simulink library "tqr"  (R2021b)
settings: Solver=VariableStepAuto  StartTime=0.0  StopTime=10.0  RelTol=1e-3
undefined symbols (not defined in the file or in its folder): ATQR_AltRDCActiveFEDUInc_X_pct, ATQR_AltRDCActiveFEDUInc_Y_enum, ATQR_AltRDCActiveFEDUTs_X_pct, ATQR_AltRDCActiveFEDUTs_Y_enum, ATQR_AltRDCActiveREDUInc_X_pct, ATQR_AltRDCActiveREDUInc_Y_enum, ATQR_AltRDCActiveREDUTs_X_pct, ATQR_AltRDCActiveREDUTs_Y_enum, ATQR_CreepFEDUTqIncSR_X_rpm, ATQR_CreepFEDUTqIncSR_Y_Nm, ATQR_CreepFEDUTs_X_rpm, ATQR_CreepFEDUTs_Y_Nm, ATQR_EcoTqFrIncGain_X_Nm, ATQR_EcoTqFrIncGain_Y_pct, ATQR_EcoTqRrIncGain_X_Nm, ATQR_EcoTqRrIncGain_Y_pct, ATQR_EL1FEDUTqDecSR_Y_Nm, ATQR_EL1FEDUTqIncSR_X_rpm, ATQR_EL1FEDUTqIncSR_Y_pct, ATQR_EL1FEDUTs_X_rpm, ATQR_EL1FEDUTs_Y_Nm, ATQR_EL1REDUTqDecSR_Y_Nm, ATQR_EL1REDUTs_Y_Nm, ATQR_FEDUEL1RegenTs_X_rpm, ATQR_FEDUTIPOutTs_X_rpm, ATQR_FrNegRateLimitIncN_X_rpm, ATQR_FrNegRateLimitIncN_Y_Nm, ATQR_FrPosRateLimitIncN_X_rpm, ATQR_FrPosRateLimitIncN_Y_Nm, ATQR_FShaftSpdTqLimCoe_X_rpm, ATQR_FTimerTqLimCoe_X_s, ATQR_FTqZeroTransUpBoundN_X_rpm, ATQR_NL1FEDUTqDecSR_Y_Nm, ATQR_NL1FEDUTqIncSR_X_rpm, ATQR_NL1FEDUTqIncSR_Y_pct, ATQR_NL1FEDUTs_X_rpm, ATQR_NL1FEDUTs_Y_Nm, ATQR_NL1REDUTqDecSR_Y_Nm, ATQR_NL1REDUTs_Y_Nm, ATQR_NormalTqFrIncGain_X_Nm, ATQR_NormalTqFrIncGain_Y_pct, ATQR_NormalTqRrIncGain_X_Nm, ATQR_NormalTqRrIncGain_Y_pct, ATQR_RrNegRateLimitIncN_X_rpm, ATQR_RrNegRateLimitIncN_Y_Nm, ATQR_RrPosRateLimitIncN_X_rpm, ATQR_RrPosRateLimitIncN_Y_Nm, ATQR_RShaftSpdTqLimCoe_X_rpm, ATQR_RTimerTqLimCoe_X_s, ATQR_SL1FEDUTqDecSR_Y_Nm, ATQR_SL1FEDUTqIncSR_X_rpm, ATQR_SL1FEDUTqIncSR_Y_pct, ATQR_SL1FEDUTs_X_rpm, ATQR_SL1FEDUTs_Y_Nm, ATQR_SL1REDUTqDecSR_Y_Nm, ATQR_SL1REDUTs_Y_Nm, ATQR_SportTqFrIncGain_X_Nm, ATQR_SportTqFrIncGain_Y_pct, ATQR_SportTqRrIncGain_X_Nm, ATQR_SportTqRrIncGain_Y_pct ... (+269)
libraries: hcu_lib x15, simulink x13, $bdroot x3
(part 3 of 9)

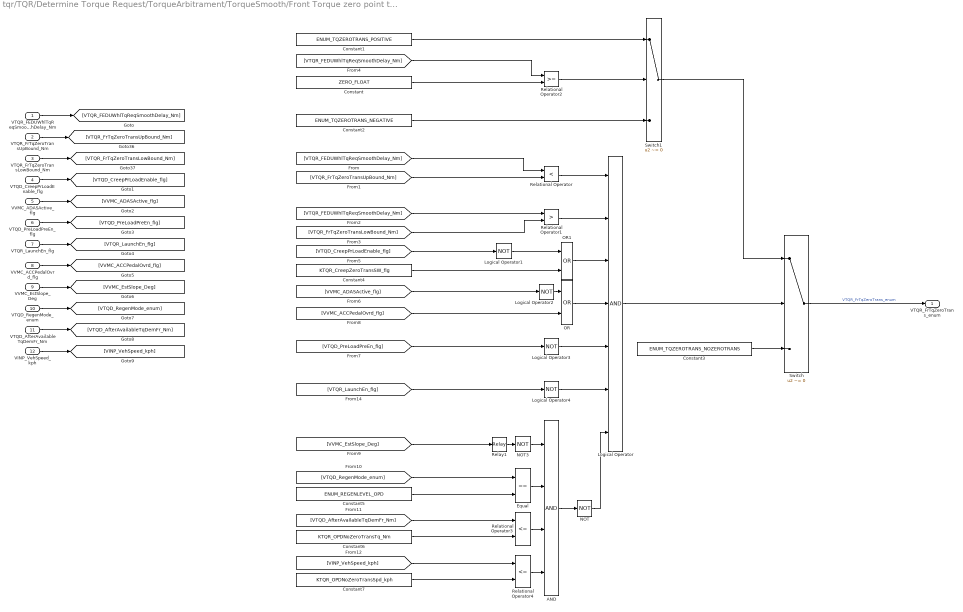
== system tqr/TQR/Determine Torque Request/TorqueArbitrament/TorqueSmooth/Front Torque zero point transfer status determination  ==
  VTQR_FEDUWhlTqReqSmoothDelay_Nm : Inport
  VTQR_FrTqZeroTransUpBound_Nm : Inport  Port=2
  VTQR_FrTqZeroTransLowBound_Nm : Inport  Port=3
  VTQD_CreepPrLoadEnable_flg : Inport  Port=4
  VVMC_ADASActive_flg : Inport  Port=5
  VTQD_PreLoadPreEn_flg : Inport  Port=6
  VTQR_LaunchEn_flg : Inport  Port=7
  VVMC_ACCPedalOvrd_flg : Inport  Port=8
  VVMC_EstSlope_Deg : Inport  Port=9
  VTQD_RegenMode_enum : Inport  Port=10
  VTQD_AfterAvailableTqDemFr_Nm : Inport  Port=11
  VINP_VehSpeed_kph : Inport  Port=12
  AND : Logic  Inputs=4  AllPortsSameDT=off  OutDataTypeStr=boolean
  Constant : Constant  Value=ZERO_FLOAT
  Constant1 : Constant  Value=ENUM_TQZEROTRANS_POSITIVE
  Constant2 : Constant  Value=ENUM_TQZEROTRANS_NEGATIVE
  Constant3 : Constant  Value=ENUM_TQZEROTRANS_NOZEROTRANS
  Constant4 : Constant  Value=KTQR_CreepZeroTransSW_flg
  Constant5 : Constant  Value=ENUM_REGENLEVEL_OPD
  Constant6 : Constant  Value=KTQR_OPDNoZeroTransTq_Nm
  Constant7 : Constant  Value=KTQR_OPDNoZeroTransSpd_kph
  Equal : RelationalOperator  Operator===  OutDataTypeStr=boolean  RndMeth=Simplest
  Logical Operator : Logic  Inputs=7  AllPortsSameDT=off  OutDataTypeStr=boolean
  Logical Operator{1..4} (4 alike) : Logic  Operator=NOT  AllPortsSameDT=off  OutDataTypeStr=boolean
  NOT : Logic  Operator=NOT  AllPortsSameDT=off  OutDataTypeStr=boolean
  NOT3 : Logic  Operator=NOT  AllPortsSameDT=off  OutDataTypeStr=boolean
  OR : Logic  Operator=OR  AllPortsSameDT=off  OutDataTypeStr=boolean
  OR1 : Logic  Operator=OR  AllPortsSameDT=off  OutDataTypeStr=boolean
  Relational Operator : RelationalOperator  Operator=<  OutDataTypeStr=boolean  RndMeth=Simplest
  Relational Operator1 : RelationalOperator  Operator=>  OutDataTypeStr=boolean  RndMeth=Simplest
  Relational Operator2 : RelationalOperator  OutDataTypeStr=boolean  RndMeth=Simplest
  Relational Operator3 : RelationalOperator  Operator=<=  OutDataTypeStr=boolean  RndMeth=Simplest
  Relational Operator4 : RelationalOperator  Operator=<=  OutDataTypeStr=boolean  RndMeth=Simplest
  Relay1 : Relay  OnSwitchValue=KTQD_OPDHoldGradeUp_Deg  OffSwitchValue=KTQD_OPDHoldGradeDown_Deg  OutDataTypeStr=boolean
  Switch : Switch  Criteria=u2 ~= 0
  Switch1 : Switch  Criteria=u2 ~= 0
  VTQR_FrTqZeroTrans_enum : Outport
  wires:
  VTQR_FEDUWhlTqReqSmoothDelay_Nm/1 -> [VTQR_FEDUWhlTqReqSmoothDelay_Nm]
  VTQR_FrTqZeroTransUpBound_Nm/1 -> [VTQR_FrTqZeroTransUpBound_Nm]
  VTQR_FrTqZeroTransLowBound_Nm/1 -> [VTQR_FrTqZeroTransLowBound_Nm]
  VTQD_CreepPrLoadEnable_flg/1 -> [VTQD_CreepPrLoadEnable_flg]
  VVMC_ADASActive_flg/1 -> [VVMC_ADASActive_flg]
  VTQD_PreLoadPreEn_flg/1 -> [VTQD_PreLoadPreEn_flg]
  VTQR_LaunchEn_flg/1 -> [VTQR_LaunchEn_flg]
  VVMC_ACCPedalOvrd_flg/1 -> [VVMC_ACCPedalOvrd_flg]
  Logical Operator2/1 -> OR/1
  [VTQR_LaunchEn_flg] -> Logical Operator4/1
  Relational Operator1/1 -> Logical Operator/2
  Relational Operator2/1 -> Switch1/2
  [VTQR_FrTqZeroTransLowBound_Nm] -> Relational Operator1/2
  OR/1 -> Logical Operator/4
  [VVMC_ACCPedalOvrd_flg] -> OR/2
  Logical Operator/1 -> Switch/2
  Logical Operator4/1 -> Logical Operator/6
  [VTQR_FEDUWhlTqReqSmoothDelay_Nm] -> Relational Operator2/1
  [VVMC_ADASActive_flg] -> Logical Operator2/1
  Switch1/1 -> Switch/1
  Logical Operator3/1 -> Logical Operator/5
  [VTQR_FEDUWhlTqReqSmoothDelay_Nm] -> Relational Operator/1
  Constant3/1 -> Switch/3
  [VTQD_PreLoadPreEn_flg] -> Logical Operator3/1
  [VTQD_CreepPrLoadEnable_flg] -> Logical Operator1/1
  Constant2/1 -> Switch1/3
  Constant1/1 -> Switch1/1
  Relational Operator/1 -> Logical Operator/1
  [VTQR_FrTqZeroTransUpBound_Nm] -> Relational Operator/2
  [VTQR_FEDUWhlTqReqSmoothDelay_Nm] -> Relational Operator1/1
  Constant/1 -> Relational Operator2/2
  Switch/1 -> VTQR_FrTqZeroTrans_enum/1  "VTQR_FrTqZeroTrans_enum"
  OR1/1 -> Logical Operator/3
  Logical Operator1/1 -> OR1/1
  Constant4/1 -> OR1/2
  Constant6/1 -> Relational Operator3/2
  NOT3/1 -> AND/1
  Constant7/1 -> Relational Operator4/2
  NOT/1 -> Logical Operator/7
  Relay1/1 -> NOT3/1
  Relational Operator3/1 -> AND/3
  Relational Operator4/1 -> AND/4
  Equal/1 -> AND/2
  Constant5/1 -> Equal/2
  AND/1 -> NOT/1
  [VVMC_EstSlope_Deg] -> Relay1/1
  [VTQD_RegenMode_enum] -> Equal/1
  [VTQD_AfterAvailableTqDemFr_Nm] -> Relational Operator3/1
  [VINP_VehSpeed_kph] -> Relational Operator4/1
  VINP_VehSpeed_kph/1 -> [VINP_VehSpeed_kph]
  VTQD_AfterAvailableTqDemFr_Nm/1 -> [VTQD_AfterAvailableTqDemFr_Nm]
  VTQD_RegenMode_enum/1 -> [VTQD_RegenMode_enum]
  VVMC_EstSlope_Deg/1 -> [VVMC_EstSlope_Deg]

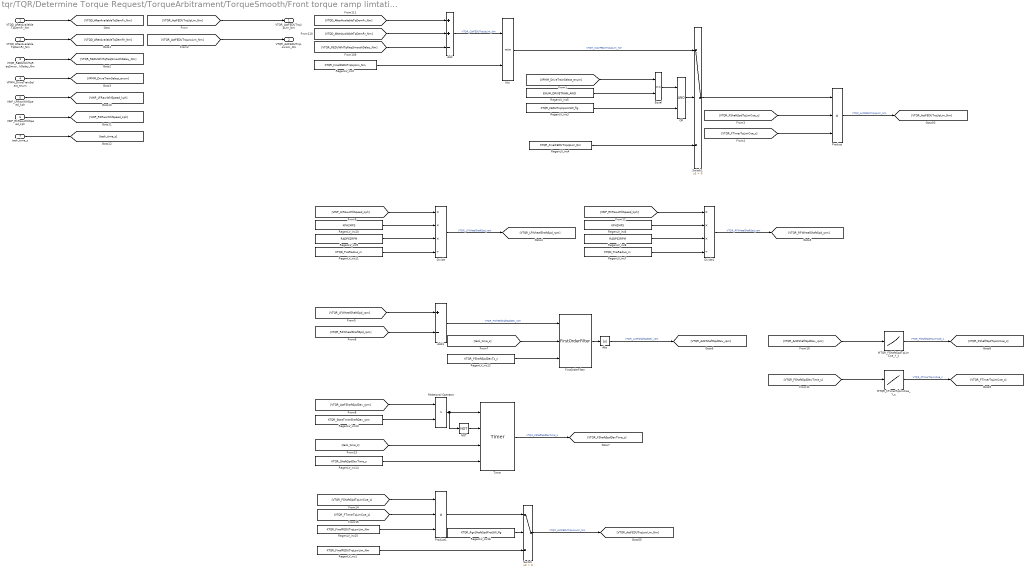
== system tqr/TQR/Determine Torque Request/TorqueArbitrament/TorqueSmooth/Front torque ramp limtation and determination ==
  VTQD_AfterAvailableTqDemFr_Nm : Inport
  VTQD_AfterAvailableTqDemRr_Nm : Inport  Port=2
  VTQR_REDUWhlTqReqSmoothDelay_Nm : Inport  Port=3
  VPMM_DriveTrainSelect_enum : Inport  Port=4
  VINP_LFRawWhlSpeed_kph : Inport  Port=5
  VINP_RFRawWhlSpeed_kph : Inport  Port=6
  task_time_s : Inport  Port=7
  Abs : Abs
  Add : Sum  Inputs=++-
  Add1 : Sum  Inputs=+-
  Divide : Product  Inputs=***/
  Divide1 : Product  Inputs=***/
  Equal : RelationalOperator  Operator===  OutDataTypeStr=boolean  RndMeth=Simplest
  FirstOrderFilter : hcu_lib/Basic_Blocks/FirstOrderFilter
  MTQR_FShaftSpdTqLimCoe_Y_c : Lookup_n-D  NumberOfTableDimensions=1  BreakpointsForDimension1=ATQR_FShaftSpdTqLimCoe_X_rpm  Table=MTQR_FShaftSpdTqLimCoe_Y_c  InternalRulePriority=Speed  RndMeth=Simplest  InputSameDT=on
  MTQR_FTimerTqLimCoe_Y_c : Lookup_n-D  NumberOfTableDimensions=1  BreakpointsForDimension1=ATQR_FTimerTqLimCoe_X_s  Table=MTQR_FTimerTqLimCoe_Y_c  InternalRulePriority=Speed  RndMeth=Simplest  InputSameDT=on
  Min : MinMax  Inputs=2
  NOT : Logic  Operator=NOT  AllPortsSameDT=off  OutDataTypeStr=boolean
  OR : Logic  AllPortsSameDT=off  OutDataTypeStr=boolean
  Product : Product  Inputs=3
  Product1 : Product  Inputs=3
  RegenLV_inc1 : Constant  Value=KTQR_FinalFEDUTrqLowLim_Nm  OutDataTypeStr=single
  RegenLV_inc10 : Constant  Value=KPH2MPS  OutDataTypeStr=single
  RegenLV_inc11 : Constant  Value=KTQD_TireRadius_m  OutDataTypeStr=single
  RegenLV_inc12 : Constant  Value=KTQR_FShaftSpdDevTs_c  OutDataTypeStr=single
  RegenLV_inc13 : Constant  Value=KTQR_StartTimerShaftDev_rpm  OutDataTypeStr=single
  RegenLV_inc14 : Constant  Value=KTQR_ShaftSpdDevTime_s  OutDataTypeStr=single
  RegenLV_inc15 : Constant  Value=KTQR_FinalFEDUTrqLowLim_Nm  OutDataTypeStr=single
  RegenLV_inc16 : Constant  Value=KTQR_RgnShaftSpdProtSW_flg  OutDataTypeStr=single
  RegenLV_inc2 : Constant  Value=KTQR_FinalFEDUTrqUpLim_Nm  OutDataTypeStr=single
  RegenLV_inc3 : Constant  Value=KTQR_FEDUTrqUpLimSW_flg  OutDataTypeStr=single
  RegenLV_inc4 : Constant  Value=KTQR_FinalFEDUTrqUpLim_Nm  OutDataTypeStr=single
  RegenLV_inc5 : Constant  Value=ENUM_DRIVETRAIN_AWD  OutDataTypeStr=single
  RegenLV_inc6 : Constant  Value=KPH2MPS  OutDataTypeStr=single
  RegenLV_inc7 : Constant  Value=KTQD_TireRadius_m  OutDataTypeStr=single
  RegenLV_inc8 : Constant  Value=RADPS2RPM  OutDataTypeStr=single
  RegenLV_inc9 : Constant  Value=RADPS2RPM  OutDataTypeStr=single
  Relational Operator : RelationalOperator  Operator=>  OutDataTypeStr=boolean  RndMeth=Simplest
  Switch : Switch  Criteria=u2 > Threshold
  Switch1 : Switch  Criteria=u2 > Threshold
  Timer : hcu_lib/Basic_Blocks/Timer
  VTQR_ActFEDUTrqUpLim_Nm : Outport
  VTQR_ActFEDUTrqLowLim_Nm : Outport  Port=2
  wires:
  Add/1 -> Min/1  "VTQR_CalFEDUTrqUpLim_Nm"
  RegenLV_inc2/1 -> Min/2
  Min/1 -> Switch1/1  "VTQR_CoorFEDUTrqUpLim_Nm"
  [VTQD_AfterAvailableTqDemFr_Nm] -> Add/1
  [VTQD_AfterAvailableTqDemRr_Nm] -> Add/2
  RegenLV_inc4/1 -> Switch1/3
  VTQD_AfterAvailableTqDemFr_Nm/1 -> [VTQD_AfterAvailableTqDemFr_Nm]
  VTQD_AfterAvailableTqDemRr_Nm/1 -> [VTQD_AfterAvailableTqDemRr_Nm]
  VTQR_REDUWhlTqReqSmoothDelay_Nm/1 -> [VTQR_REDUWhlTqReqSmoothDelay_Nm]
  VPMM_DriveTrainSelect_enum/1 -> [VPMM_DriveTrainSelect_enum]
  [VTQR_REDUWhlTqReqSmoothDelay_Nm] -> Add/3
  [VTQR_ActFEDUTrqLowLim_Nm] -> VTQR_ActFEDUTrqLowLim_Nm/1
  [VTQR_ActFEDUTrqUpLim_Nm] -> VTQR_ActFEDUTrqUpLim_Nm/1
  [VPMM_DriveTrainSelect_enum] -> Equal/1
  RegenLV_inc5/1 -> Equal/2
  RegenLV_inc3/1 -> OR/2
  OR/1 -> Switch1/2
  Equal/1 -> OR/1
  [VTQR_FShaftSpdDevTime_s] -> MTQR_FTimerTqLimCoe_Y_c/1
  MTQR_FTimerTqLimCoe_Y_c/1 -> [VTQR_FTimerTqLimCoe_c]  "VTQR_FTimerTqLimCoe_c"
  Timer/1 -> [VTQR_FShaftSpdDevTime_s]  "VTQR_FShaftSpdDevTime_s"
  [VTQR_RFWheelShaftSpd_rpm] -> Add1/2
  [VTQR_ActFShaftSpdDev_rpm] -> Relational Operator/1
  Relational Operator/1 -> Timer/1, NOT/1
  MTQR_FShaftSpdTqLimCoe_Y_c/1 -> [VTQR_FShaftSpdTqLimCoe_c]  "VTQR_FShaftSpdTqLimCoe_c"
  RegenLV_inc12/1 -> FirstOrderFilter/3
  RegenLV_inc14/1 -> Timer/4
  [task_time_s] -> Timer/3
  RegenLV_inc9/1 -> Divide/3
  RegenLV_inc6/1 -> Divide1/2
  RegenLV_inc10/1 -> Divide/2
  RegenLV_inc13/1 -> Relational Operator/2
  RegenLV_inc8/1 -> Divide1/3
  [VTQR_ActFShaftSpdDev_rpm] -> MTQR_FShaftSpdTqLimCoe_Y_c/1
  Divide/1 -> [VTQR_LFWheelShaftSpd_rpm]  "VTQR_LFWheelShaftSpd_rpm"
  RegenLV_inc7/1 -> Divide1/4
  Divide1/1 -> [VTQR_RFWheelShaftSpd_rpm]  "VTQR_RFWheelShaftSpd_rpm"
  RegenLV_inc11/1 -> Divide/4
  Add1/1 -> FirstOrderFilter/1  "VTQR_FWheelShaftSpdDev_rpm"
  NOT/1 -> Timer/2
  [VTQR_LFWheelShaftSpd_rpm] -> Add1/1
  [task_time_s] -> FirstOrderFilter/2
  Abs/1 -> [VTQR_ActFShaftSpdDev_rpm]  "VTQR_ActFShaftSpdDev_rpm"
  FirstOrderFilter/1 -> Abs/1
  [VINP_LFRawWhlSpeed_kph] -> Divide/1
  [VINP_RFRawWhlSpeed_kph] -> Divide1/1
  VINP_RFRawWhlSpeed_kph/1 -> [VINP_RFRawWhlSpeed_kph]
  task_time_s/1 -> [task_time_s]
  VINP_LFRawWhlSpeed_kph/1 -> [VINP_LFRawWhlSpeed_kph]
  Switch1/1 -> Product/1
  [VTQR_FTimerTqLimCoe_c] -> Product/3
  [VTQR_FShaftSpdTqLimCoe_c] -> Product/2
  Product/1 -> [VTQR_ActFEDUTrqUpLim_Nm]  "VTQR_ActFEDUTrqUpLim_Nm"
  Product1/1 -> Switch/1
  RegenLV_inc16/1 -> Switch/2
  RegenLV_inc1/1 -> Switch/3
  Switch/1 -> [VTQR_ActFEDUTrqLowLim_Nm]  "VTQR_ActFEDUTrqLowLim_Nm"
  RegenLV_inc15/1 -> Product1/3
  [VTQR_FShaftSpdTqLimCoe_c] -> Product1/1
  [VTQR_FTimerTqLimCoe_c] -> Product1/2

== system tqr/TQR/Determine Torque Request/TorqueArbitrament/TorqueSmooth/Front wheel first order filter input torque command determination ==
  VTQR_FrTqZeroTrans_enum : Inport
  VTQR_FrTqZeroTransUpBound_Nm : Inport  Port=2
  VTQR_FrTqZeroTransLowBound_Nm : Inport  Port=3
  VTQD_AfterAvailableTqDemFr_Nm : Inport  Port=4
  VTQR_FrFirstOrderOutTqDelay_Nm : Inport  Port=5
  VTQR_FrGearChange_flg : Inport  Port=6
  VTQR_RampTqCMDGain_c : Inport  Port=7
  AND : Logic  AllPortsSameDT=off  OutDataTypeStr=boolean
  Constant1 : Constant  Value=ZERO_FLOAT
  Constant2 : Constant  Value=KTQR_GearChangeTqSW_flg
  Constant3 : Constant  Value=ENUM_TQZEROTRANS_NOZEROTRANS
  Constant4 : Constant  Value=KTQR_NewRampArchSW_flg
  Constant5 : Constant  Value=ONE_FLOAT
  Product : Product
  Relational Operator : RelationalOperator  Operator===  OutDataTypeStr=boolean  RndMeth=Simplest
  Relational Operator1 : RelationalOperator  OutDataTypeStr=boolean  RndMeth=Simplest
  Relational Operator2 : RelationalOperator  Operator=<=  OutDataTypeStr=boolean  RndMeth=Simplest
  Switch : Switch  Criteria=u2 ~= 0
  Switch1 : Switch  Criteria=u2 ~= 0
  Switch2 : Switch  Criteria=u2 ~= 0
  Switch3 : Switch  Criteria=u2 > Threshold
  Switch4 : Switch  Criteria=u2 > Threshold
  VTQR_FrFirstOrderInpTq_Nm : Outport
  wires:
  [VTQR_FrTqZeroTrans_enum] -> Relational Operator/1
  Constant3/1 -> Relational Operator/2
  Relational Operator/1 -> Switch/2
  Switch1/1 -> Switch/3
  Relational Operator1/1 -> Switch1/2
  [VTQR_FrFirstOrderOutTqDelay_Nm] -> Relational Operator1/1
  [VTQR_FrTqZeroTransUpBound_Nm] -> Relational Operator1/2
  [VTQR_FrTqZeroTransUpBound_Nm] -> Switch1/1
  Switch3/1 -> VTQR_FrFirstOrderInpTq_Nm/1  "VTQR_FrFirstOrderInpTq_Nm"
  [VTQR_FrTqZeroTransLowBound_Nm] -> Switch2/1
  Switch2/1 -> Switch1/3
  [VTQR_FrFirstOrderOutTqDelay_Nm] -> Relational Operator2/1
  [VTQR_FrTqZeroTransLowBound_Nm] -> Relational Operator2/2
  Relational Operator2/1 -> Switch2/2
  [VTQR_FrActRampTqDem_Nm] -> Switch2/3
  VTQR_FrTqZeroTransLowBound_Nm/1 -> [VTQR_FrTqZeroTransLowBound_Nm]
  VTQR_FrTqZeroTrans_enum/1 -> [VTQR_FrTqZeroTrans_enum]
  VTQR_FrFirstOrderOutTqDelay_Nm/1 -> [VTQR_FrFirstOrderOutTqDelay_Nm]
  VTQD_AfterAvailableTqDemFr_Nm/1 -> [VTQD_AfterAvailableTqDemFr_Nm]
  VTQR_FrTqZeroTransUpBound_Nm/1 -> [VTQR_FrTqZeroTransUpBound_Nm]
  VTQR_FrGearChange_flg/1 -> [VTQR_FrGearChange_flg]
  Constant1/1 -> Switch3/1
  Constant2/1 -> AND/2
  [VTQR_FrGearChange_flg] -> AND/1
  AND/1 -> Switch3/2
  Switch/1 -> Switch3/3
  VTQR_RampTqCMDGain_c/1 -> [VTQR_RampTqCMDGain_c]
  Switch4/1 -> Product/2
  [VTQR_RampTqCMDGain_c] -> Switch4/1
  Constant4/1 -> Switch4/2
  Constant5/1 -> Switch4/3
  Product/1 -> [VTQR_FrActRampTqDem_Nm]  "VTQR_FrActRampTqDem_Nm"
  [VTQR_FrActRampTqDem_Nm] -> Switch/1
  [VTQD_AfterAvailableTqDemFr_Nm] -> Product/1

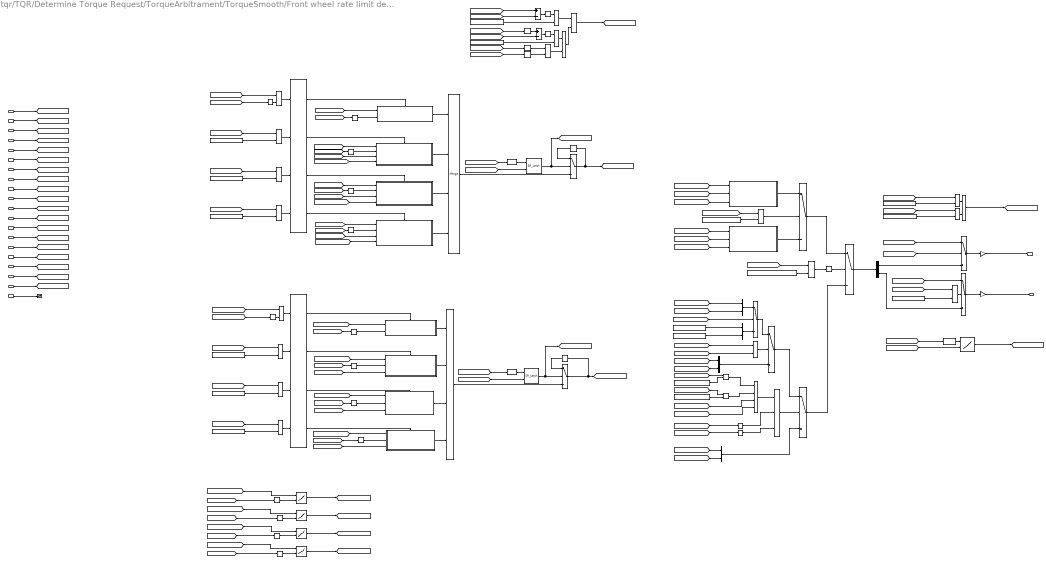
== system tqr/TQR/Determine Torque Request/TorqueArbitrament/TorqueSmooth/Front wheel rate limit determination ==
  VTQR_FrTqZeroTrans_enum : Inport
  VTQD_TqSourceFr_enum : Inport  Port=2
  VTQD_TqTargetShaftSpd_rpm : Inport  Port=3
  VTQD_LimpHomeAct_flg : Inport  Port=4
  VTQR_EVDriveMode_enum : Inport  Port=5
  VDHP_ActAPSPosn_pct : Inport  Port=6
  VTQR_FEDUWhlTqReqSmoothDelay_Nm : Inport  Port=7
  VTQD_EVDriveModeValid_flg : Inport  Port=8
  VTQD_RegenMode_enum : Inport  Port=9
  VVMC_ACCPedalOvrd_flg : Inport  Port=10
  VVMC_CCPedalOvrd_flg : Inport  Port=11
  VTQD_CreepPrLoadEnable_flg : Inport  Port=12
  VTQD_RegenTqLimitEn_flg : Inport  Port=13
  VTQD_RDCActive_enum : Inport  Port=14
  VTQD_PreLoadPreEn_flg : Inport  Port=15
  VTQR_NoABSFEDUWhlTqReq_Nm : Inport  Port=16
  VTQR_RampFEDUWhlTqReq_Nm : Inport  Port=17
  VTQR_FrFirstOrderInpTq_Nm : Inport  Port=18
  VVMC_ActMaxSlideRate_pct : Inport  Port=19
  VTQD_PedAccTqEn_flg : Inport  Port=20
  AND : Logic  AllPortsSameDT=off  OutDataTypeStr=boolean
  AND1 : Logic  Inputs=3  AllPortsSameDT=off  OutDataTypeStr=boolean
  AND2 : Logic  AllPortsSameDT=off  OutDataTypeStr=boolean
  AND4 : Logic  AllPortsSameDT=off  OutDataTypeStr=boolean
  Abs{,1..4,10..13,15..17,43,47} (14 alike) : Abs
  Add : Sum  Inputs=+-
  Add1 : Sum  Inputs=+-
  Constant1 : Constant  Value=ENUM_TQZEROTRANS_NOZEROTRANS
  Constant10 : Constant  Value=KTQR_PreLoadTqIncSR_Nm
  Constant11 : Constant  Value=KTQR_DriveModeCMDTqDev_Nm
  Constant12 : Constant  Value=KTQR_ARegenLatchEnTq_Nm
  Constant13 : Constant  Value=KTQR_PreLoadTqDecSR_Nm
  Constant14 : Constant  Value=ENUM_DRIVEMODE_ECO
  Constant15 : Constant  Value=ENUM_DRIVEMODE_NRM
  Constant17 : Constant  Value=ENUM_DRIVEMODE_SPORT
  Constant2 : Constant  Value=ENUM_RDCACTSTA_NOREQUEST
  Constant3 : Constant  Value=ENUM_TQSOURCE_CC
  Constant34 : Constant  Value=ENUM_TQSOURCE_ADAS
  Constant4 : Constant  Value=ENUM_TQZEROTRANS_POSITIVE
  Constant5 : Constant  Value=KTQR_DriveModeChangeTq_Nm
  Constant6 : Constant  Value=KTQR_RegenTqLimitDecSW_flg
  Constant7 : Constant  Value=ENUM_DRIVEMODE_ECO
  Constant8 : Constant  Value=ENUM_DRIVEMODE_NRM
  Constant9 : Constant  Value=ENUM_DRIVEMODE_SPORT
  Data Type Conversion : DataTypeConversion  OutDataTypeStr=single
  Delay{,1..4} (5 alike) : Delay  DelayLength=1
  Demux : Demux  Outputs=2
  Detect Change : simulink/Logic and Bit Operations/Detect Change  vinit=0  OutDataTypeStr=boolean
  Detect Change1 : simulink/Logic and Bit Operations/Detect Change  vinit=0  OutDataTypeStr=boolean
  Equal{5..6,8,12..13,15} (6 alike) : RelationalOperator  Operator===  OutDataTypeStr=boolean  RndMeth=Simplest
  Equal2 : RelationalOperator  Operator=~=  OutDataTypeStr=boolean  RndMeth=Simplest
  Gain : Gain
  Gain1 : Gain
  If1 : If  NumInputs=4  IfExpression=u1~= 0  ElseIfExpressions=u2 ~= 0, u3 ~= 0,u4 ~= 0  ShowElse=off
  If2 : If  NumInputs=4  IfExpression=u1~= 0  ElseIfExpressions=u2 ~= 0, u3 ~= 0,u4 ~= 0  ShowElse=off
  Logical Operator1 : Logic  Operator=NOT  AllPortsSameDT=off  OutDataTypeStr=boolean
  Logical Operator14 : Logic  Operator=OR  Inputs=4  AllPortsSameDT=off  OutDataTypeStr=boolean
  Logical Operator4 : Logic  Operator=OR  AllPortsSameDT=off  OutDataTypeStr=boolean
  Logical Operator5 : Logic  Operator=NOT  AllPortsSameDT=off  OutDataTypeStr=boolean
  Logical Operator6 : Logic  Operator=OR  AllPortsSameDT=off  OutDataTypeStr=boolean
  Logical Operator7 : Logic  Operator=NOT  AllPortsSameDT=off  OutDataTypeStr=boolean
  MTQR_AltRDCActiveFEDUInc_Z_Nm : Lookup_n-D  BreakpointsForDimension1=ATQR_AltRDCActiveFEDUInc_Y_enum  BreakpointsForDimension2=ATQR_AltRDCActiveFEDUInc_X_pct  Table=MTQR_AltRDCActiveFEDUInc_Z_Nm  TableDataTypeStr=Inherit: Inherit from 'Table data'  ExtrapMethod=Clip  InternalRulePriority=Speed  RndMeth=Simplest  InputSameDT=on
      settings: InputPortMap=u0,u1
  MTQR_CreepFEDUTqDecSR_Z_Nm : Lookup_n-D  BreakpointsForDimension1=ATQR_CreepFEDUTqIncSR_Y_Nm  BreakpointsForDimension2=ATQR_CreepFEDUTqIncSR_X_rpm  Table=MTQR_CreepFEDUTqDecSR_Z_Nm  ExtrapMethod=Clip  InternalRulePriority=Speed  RndMeth=Simplest  InputSameDT=on
      settings: InputPortMap=u0,u1
  MTQR_CreepFEDUTqIncSR_Z_Nm : Lookup_n-D  BreakpointsForDimension1=ATQR_CreepFEDUTqIncSR_Y_Nm  BreakpointsForDimension2=ATQR_CreepFEDUTqIncSR_X_rpm  Table=MTQR_CreepFEDUTqIncSR_Z_Nm  ExtrapMethod=Clip  InternalRulePriority=Speed  RndMeth=Simplest  InputSameDT=on
      settings: InputPortMap=u0,u1
  MTQR_VMCFEDUTqDecSR_Z_Nm : Lookup_n-D  BreakpointsForDimension1=ATQR_VMCFEDUTqIncSR_Y_Nm  BreakpointsForDimension2=ATQR_VMCFEDUTqIncSR_X_rpm  Table=MTQR_VMCFEDUTqDecSR_Z_Nm  ExtrapMethod=Clip  InternalRulePriority=Speed  RndMeth=Simplest  InputSameDT=on
      settings: InputPortMap=u0,u1
  MTQR_VMCFEDUTqIncSR_Z_Nm : Lookup_n-D  BreakpointsForDimension1=ATQR_VMCFEDUTqIncSR_Y_Nm  BreakpointsForDimension2=ATQR_VMCFEDUTqIncSR_X_rpm  Table=MTQR_VMCFEDUTqIncSR_Z_Nm  ExtrapMethod=Clip  InternalRulePriority=Speed  RndMeth=Simplest  InputSameDT=on
      settings: InputPortMap=u0,u1
  Merge1 : Merge  Inputs=4
  Merge2 : Merge  Inputs=4
  Mux{1..4} (4 alike) : Mux  Inputs=2
  NOT : Logic  Operator=NOT  AllPortsSameDT=off  OutDataTypeStr=boolean
  NOT1 : Logic  Operator=NOT  AllPortsSameDT=off  OutDataTypeStr=boolean
  Negative Rate limit Determination : Subsystem  TreatAsAtomicUnit=on
  OR : Logic  Operator=OR  AllPortsSameDT=off  OutDataTypeStr=boolean
  OR2 : Logic  Operator=OR  AllPortsSameDT=off  OutDataTypeStr=boolean
  OR3 : Logic  Operator=OR  AllPortsSameDT=off  OutDataTypeStr=boolean
  Positive Rate limit Determination : Subsystem  TreatAsAtomicUnit=on
  Relational Operator{,1,3..4} (4 alike) : RelationalOperator  Operator===  OutDataTypeStr=boolean  RndMeth=Simplest
  Relational Operator2 : RelationalOperator  Operator=<=  OutDataTypeStr=boolean  RndMeth=Simplest
  Relational Operator5 : RelationalOperator  Operator=<  OutDataTypeStr=boolean  RndMeth=Simplest
  Relational Operator6 : RelationalOperator  OutDataTypeStr=boolean  RndMeth=Simplest
  SR_Latch1 : hcu_lib/Basic_Blocks/SR_Latch
  SR_Latch2 : hcu_lib/Basic_Blocks/SR_Latch
  Switch{,4..7} (5 alike) : Switch  Criteria=u2 > Threshold
  Switch1 : Switch  Criteria=u2 ~= 0  Threshold=0.5
  Switch13 : Switch  Criteria=u2 ~= 0
  Switch2 : Switch  Criteria=u2 ~= 0
  Switch3 : Switch  Criteria=u2 ~= 0  Threshold=0.5
  Terminator : Terminator
  VTQR_ECOFEDURateLimitDec_Nm : Subsystem  TreatAsAtomicUnit=on
  VTQR_ECOFEDURateLimitInc_Nm : Subsystem  TreatAsAtomicUnit=on
  VTQR_LHMFEDURateLimitDec_Nm : Subsystem  AncestorBlock=tqr/TQR/Determine Torque Request/TorqueArbitrament/TorqueSmooth/VTQR_LHMFEDURateLimitDec_Nm  TreatAsAtomicUnit=on
  VTQR_LHMFEDURateLimitInc_Nm : Subsystem  AncestorBlock=tqr/TQR/Determine Torque Request/TorqueArbitrament/TorqueSmooth/VTQR_LHMFEDURateLimitInc_Nm  TreatAsAtomicUnit=on
  VTQR_NORMALFEDURateLimitDec_Nm : Subsystem  AncestorBlock=tqr/TQR/Determine Torque Request/TorqueArbitrament/TorqueSmooth/VTQR_NORMALFEDURateLimitDec_Nm  TreatAsAtomicUnit=on
  VTQR_NORMALFEDURateLimitInc_Nm : Subsystem  TreatAsAtomicUnit=on
  VTQR_SPORTFEDURateLimitDec_Nm : Subsystem  AncestorBlock=tqr/TQR/Determine Torque Request/TorqueArbitrament/TorqueSmooth/VTQR_SPORTFEDURateLimitDec_Nm  TreatAsAtomicUnit=on
  VTQR_SPORTFEDURateLimitInc_Nm : Subsystem  TreatAsAtomicUnit=on
  VTQR_FrRateLimitInc_Nm : Outport
  VTQR_FrRateLimitDec_Nm : Outport  Port=2
  wires:
  VTQR_FrTqZeroTrans_enum/1 -> [VTQR_FrTqZeroTrans_enum]
  VTQD_TqSourceFr_enum/1 -> [VTQD_TqSourceFr_enum]
  AND1/1 -> Switch13/2
  Mux4/1 -> Switch13/3
  Switch13/1 -> Switch3/3
  Logical Operator7/1 -> Switch3/2
  Relational Operator/1 -> Logical Operator7/1
  Constant1/1 -> Relational Operator/2
  [VTQR_FrTqZeroTrans_enum] -> Relational Operator/1
  [VTQR_FrTqZeroTrans_enum] -> Relational Operator1/1
  Relational Operator1/1 -> Switch1/2
  Constant4/1 -> Relational Operator1/2
  Switch1/1 -> Switch3/1
  Switch3/1 -> Demux/1
  Positive Rate limit Determination/1(VTQR_PosRateLimit_mux) -> Switch1/1
  [VTQR_VMCFEDUTqIncSR_Nm] -> Mux3/1
  [VTQR_VMCFEDUTqDecSR_Nm] -> Mux3/2
  [VTQR_FEDURateLimitInc_Nm] -> Mux4/1
  [VTQR_FEDURateLimitDec_Nm] -> Mux4/2
  Switch/1 -> Gain/1
  Gain/1 -> VTQR_FrRateLimitInc_Nm/1  "VTQR_FrRateLimitInc_Nm"
  Gain1/1 -> VTQR_FrRateLimitDec_Nm/1  "VTQR_FrRateLimitDec_Nm"
  VTQD_TqTargetShaftSpd_rpm/1 -> [VTQD_TqTargetShaftSpd_rpm]
  If2/3 -> VTQR_ECOFEDURateLimitDec_Nm/Action
  Equal12/1 -> If2/3
  Equal15/1 -> If2/4
  Logical Operator6/1 -> If2/1
  MTQR_VMCFEDUTqDecSR_Z_Nm/1 -> [VTQR_VMCFEDUTqDecSR_Nm]  "VTQR_VMCFEDUTqDecSR_Nm"
  [VTQR_EVDriveMode_enum] -> Equal15/1
  Logical Operator4/1 -> If1/1
  MTQR_VMCFEDUTqIncSR_Z_Nm/1 -> [VTQR_VMCFEDUTqIncSR_Nm]  "VTQR_VMCFEDUTqIncSR_Nm"
  VTQR_LHMFEDURateLimitInc_Nm/1(VTQR_LHMFEDURateLimitInc_Nm) -> Merge1/1
  Logical Operator5/1 -> Logical Operator4/2
  If2/2 -> VTQR_NORMALFEDURateLimitDec_Nm/Action
  If1/1 -> VTQR_LHMFEDURateLimitInc_Nm/Action
  [VTQD_TqTargetShaftSpd_rpm] -> Abs10/1
  Abs16/1 -> VTQR_ECOFEDURateLimitDec_Nm/2(VTQD_TqTargetShaftSpd_rpm)  "VTQD_TqTargetShaftSpd_rpm"
  Logical Operator1/1 -> Logical Operator6/2
  If2/4 -> VTQR_SPORTFEDURateLimitDec_Nm/Action
  [VTQR_EVDriveMode_enum] -> Equal13/1
  Constant14/1 -> Equal12/2
  Constant17/1 -> Equal15/2
  [VTQR_EVDriveMode_enum] -> Equal12/1
  Equal13/1 -> If2/2
  Equal6/1 -> If1/2
  [VTQD_EVDriveModeValid_flg] -> Logical Operator5/1
  [VTQD_LimpHomeAct_flg] -> Logical Operator4/1
  Equal5/1 -> If1/3
  [VTQR_EVDriveMode_enum] -> Equal8/1
  Abs2/1 -> VTQR_LHMFEDURateLimitDec_Nm/2(VTQD_TqTargetShaftSpd_rpm)  "VTQD_TqTargetShaftSpd_rpm"
  [VTQR_EVDriveMode_enum] -> Equal6/1
  [VTQR_FEDUWhlTqReqSmoothDelay_Nm] -> VTQR_SPORTFEDURateLimitDec_Nm/1(VTQR_FEDUWhlTqReqSmoothDelay_Nm)
  Abs15/1 -> VTQR_SPORTFEDURateLimitDec_Nm/2(VTQD_TqTargetShaftSpd_rpm)  "VTQD_TqTargetShaftSpd_rpm"
  [VTQD_TqTargetShaftSpd_rpm] -> Abs15/1
  [VTQD_TqTargetShaftSpd_rpm] -> Abs2/1
  Equal8/1 -> If1/4
  Constant9/1 -> Equal8/2
  Constant8/1 -> Equal6/2
  VTQR_ECOFEDURateLimitDec_Nm/1(VTQR_ECOFEDURateLimitDec_Nm) -> Merge2/3
  Abs10/1 -> VTQR_LHMFEDURateLimitInc_Nm/2(VTQD_TqTargetShaftSpd_rpm)  "VTQD_TqTargetShaftSpd_rpm"
  Constant7/1 -> Equal5/2
  Constant15/1 -> Equal13/2
  [VTQD_TqTargetShaftSpd_rpm] -> Abs16/1
  [VTQR_FEDUWhlTqReqSmoothDelay_Nm] -> VTQR_LHMFEDURateLimitDec_Nm/1(VTQR_FEDUWhlTqReqSmoothDelay_Nm)
  [VTQD_LimpHomeAct_flg] -> Logical Operator6/1
  [VDHP_ActAPSPosn_pct] -> VTQR_LHMFEDURateLimitInc_Nm/1(VDHP_ActAPSPosn_pct)
  VTQR_LHMFEDURateLimitDec_Nm/1(VTQR_LHMFEDURateLimitDec_Nm) -> Merge2/1
  [VTQD_TqTargetShaftSpd_rpm] -> Abs17/1
  VTQR_SPORTFEDURateLimitDec_Nm/1(VTQR_SPORTFEDURateLimitDec_Nm) -> Merge2/4
  [VTQD_EVDriveModeValid_flg] -> Logical Operator1/1
  [VTQR_FEDUWhlTqReqSmoothDelay_Nm] -> VTQR_ECOFEDURateLimitDec_Nm/1(VTQR_FEDUWhlTqReqSmoothDelay_Nm)
  [VTQR_EVDriveMode_enum] -> Equal5/1
  If2/1 -> VTQR_LHMFEDURateLimitDec_Nm/Action
  VTQD_LimpHomeAct_flg/1 -> [VTQD_LimpHomeAct_flg]
  VTQR_EVDriveMode_enum/1 -> [VTQR_EVDriveMode_enum]
  VDHP_ActAPSPosn_pct/1 -> [VDHP_ActAPSPosn_pct]
  VTQR_FEDUWhlTqReqSmoothDelay_Nm/1 -> [VTQR_FEDUWhlTqReqSmoothDelay_Nm]
  VTQD_EVDriveModeValid_flg/1 -> [VTQD_EVDriveModeValid_flg]
  [VTQR_FEDUWhlTqReqSmoothDelay_Nm] -> VTQR_NORMALFEDURateLimitDec_Nm/1(VTQR_FEDUWhlTqReqSmoothDelay_Nm)
  Abs17/1 -> VTQR_NORMALFEDURateLimitDec_Nm/2(VTQD_TqTargetShaftSpd_rpm)  "VTQD_TqTargetShaftSpd_rpm"
  VTQR_NORMALFEDURateLimitDec_Nm/1(VTQR_NORMALFEDURateLimitDec_Nm) -> Merge2/2
  VTQD_RegenMode_enum/1 -> [VTQD_RegenMode_enum]
  [VTQD_RegenMode_enum] -> VTQR_NORMALFEDURateLimitDec_Nm/3(VTQD_RegenMode_enum)
  [VTQD_RegenMode_enum] -> VTQR_ECOFEDURateLimitDec_Nm/3(VTQD_RegenMode_enum)
  [VTQD_RegenMode_enum] -> VTQR_SPORTFEDURateLimitDec_Nm/3(VTQD_RegenMode_enum)
  [VTQR_FEDUWhlTqReqSmoothDelay_Nm] -> MTQR_VMCFEDUTqIncSR_Z_Nm/1
  Abs43/1 -> MTQR_VMCFEDUTqIncSR_Z_Nm/2
  Abs47/1 -> MTQR_VMCFEDUTqDecSR_Z_Nm/2
  [VTQR_FEDUWhlTqReqSmoothDelay_Nm] -> MTQR_VMCFEDUTqDecSR_Z_Nm/1
  [VTQR_FEDUWhlTqReqSmoothDelay_Nm] -> Positive Rate limit Determination/2(VTQR_FEDUWhlTqReqSmoothDelay_Nm)
  [VTQR_FEDUWhlTqReqSmoothDelay_Nm] -> Negative Rate limit Determination/2(VTQR_FEDUWhlTqReqSmoothDelay_Nm)
  VVMC_ACCPedalOvrd_flg/1 -> [VVMC_ACCPedalOvrd_flg]
  VVMC_CCPedalOvrd_flg/1 -> [VVMC_CCPedalOvrd_flg]
  Logical Operator14/1 -> AND1/1
  [VVMC_CCPedalOvrd_flg] -> NOT1/1
  Constant3/1 -> Relational Operator3/2
  [VVMC_ACCPedalOvrd_flg] -> NOT/1
  NOT/1 -> AND1/2
  NOT1/1 -> AND1/3
  [VTQD_TqSourceFr_enum] -> Relational Operator4/1
  [VTQD_TqSourceFr_enum] -> Relational Operator3/1
  Constant34/1 -> Relational Operator4/2
  Relational Operator4/1 -> Logical Operator14/2
  Relational Operator3/1 -> Logical Operator14/1
  [VTQR_EVDriveMode_enum] -> Positive Rate limit Determination/3(VTQR_EVDriveMode_enum)
  [VTQR_EVDriveMode_enum] -> Negative Rate limit Determination/3(VTQR_EVDriveMode_enum)
  Negative Rate limit Determination/1(VTQR_NegRateLimit_mux) -> Switch1/3
  [VTQD_TqTargetShaftSpd_rpm] -> Abs43/1
  [VTQD_TqTargetShaftSpd_rpm] -> Abs47/1
  [VTQD_TqTargetShaftSpd_rpm] -> Positive Rate limit Determination/1(VTQD_TqTargetShaftSpd_rpm)
  [VTQD_TqTargetShaftSpd_rpm] -> Negative Rate limit Determination/1(VTQD_TqTargetShaftSpd_rpm)
  [VTQR_FEDUWhlTqReqSmoothDelay_Nm] -> MTQR_CreepFEDUTqIncSR_Z_Nm/1
  MTQR_CreepFEDUTqIncSR_Z_Nm/1 -> [VTQR_CreepFEDUTqIncSR_Nm]  "VTQR_CreepFEDUTqIncSR_Nm"
  [VTQR_FEDUWhlTqReqSmoothDelay_Nm] -> MTQR_CreepFEDUTqDecSR_Z_Nm/1
  Abs1/1 -> MTQR_CreepFEDUTqIncSR_Z_Nm/2
  [VTQD_TqTargetShaftSpd_rpm] -> Abs3/1
  MTQR_CreepFEDUTqDecSR_Z_Nm/1 -> [VTQR_CreepFEDUTqDecSR_Nm]  "VTQR_CreepFEDUTqDecSR_Nm"
  Abs3/1 -> MTQR_CreepFEDUTqDecSR_Z_Nm/2
  [VTQD_TqTargetShaftSpd_rpm] -> Abs1/1
  [VTQR_FrRDCActRateLimitInc_flg] -> Switch/2
  Demux/1 -> Switch/3
  [VTQD_CreepPrLoadEnable_flg] -> Logical Operator14/3
  [VTQD_PreLoadPreEn_flg] -> Logical Operator14/4
  Mux3/1 -> Switch2/3
  [VTQD_CreepPrLoadEnable_flg] -> OR/1
  OR/1 -> Switch2/2
  [VTQR_CreepFEDUTqDecSR_Nm] -> Mux1/2
  [VTQD_PreLoadPreEn_flg] -> OR/2
  [VTQR_CreepFEDUTqIncSR_Nm] -> Mux1/1
  Switch2/1 -> Switch13/1
  VTQD_CreepPrLoadEnable_flg/1 -> [VTQD_CreepPrLoadEnable_flg]
  VTQD_PreLoadPreEn_flg/1 -> [VTQD_PreLoadPreEn_flg]
  VTQD_RDCActive_enum/1 -> [VTQD_RDCActive_enum]
  VTQR_NoABSFEDUWhlTqReq_Nm/1 -> [VTQR_NoABSFEDUWhlTqReq_Nm]
  VTQR_RampFEDUWhlTqReq_Nm/1 -> [VTQR_RampFEDUWhlTqReq_Nm]
  Relational Operator2/1 -> AND/1
  [VTQD_RDCActive_enum] -> Equal2/1
  Constant2/1 -> Equal2/2
  Equal2/1 -> AND/2
  [VTQR_RampFEDUWhlTqReq_Nm] -> Relational Operator2/1
  Constant12/1 -> Relational Operator2/2
  AND/1 -> [VTQR_FrRDCActRateLimitInc_flg]  "VTQR_FrRDCActRateLimitInc_flg"
  VTQR_FrFirstOrderInpTq_Nm/1 -> [VTQR_FrFirstOrderInpTq_Nm]
  [VTQR_NoABSFEDUWhlTqReq_Nm] -> Add/1
  Delay/1 -> Switch4/1
  AND4/1 -> OR2/2
  [VTQR_FrDrModIncLatch_flg] -> Delay3/1
  Delay4/1 -> OR3/2
  Relational Operator6/1 -> AND4/1
  [VTQR_FrFirstOrderInpTq_Nm] -> Add/2
  OR3/1 -> AND4/2
  [VTQR_FrDrModChangeReset_flg] -> SR_Latch1/2
  Constant11/1 -> Relational Operator6/2
  Relational Operator5/1 -> OR2/1
  Add1/1 -> Abs4/1
  [VTQR_FrFirstOrderInpTq_Nm] -> Add1/2
  Switch4/1 -> [VTQR_FEDURateLimitInc_Nm], Delay/1  "VTQR_FEDURateLimitInc_Nm"
  [VTQR_FrFirstOrderInpTq_Nm] -> Delay1/1
  [VTQR_EVDriveMode_enum] -> Detect Change/1
  Abs4/1 -> Relational Operator6/1
  Delay1/1 -> Add1/1
  Delay3/1 -> OR3/1
  OR2/1 -> [VTQR_FrDrModChangeReset_flg]  "VTQR_FrDrModChangeReset_flg"
  SR_Latch1/1 -> Switch4/2, [VTQR_FrDrModIncLatch_flg]
  Merge1/1 -> Switch4/3
  Detect Change/1 -> SR_Latch1/1
  Abs/1 -> Relational Operator5/1
  Add/1 -> Abs/1
  Constant5/1 -> Relational Operator5/2
  Merge2/1 -> Switch5/3
  [VTQR_FrDrModChangeReset_flg] -> SR_Latch2/2
  Switch5/1 -> [VTQR_FEDURateLimitDec_Nm], Delay2/1  "VTQR_FEDURateLimitDec_Nm"
  Delay2/1 -> Switch5/1
  Detect Change1/1 -> SR_Latch2/1
  [VTQR_EVDriveMode_enum] -> Detect Change1/1
  SR_Latch2/1 -> Switch5/2, [VTQR_FrDrModDecLatch_flg]
  [VTQD_RegenMode_enum] -> Data Type Conversion/1
  MTQR_AltRDCActiveFEDUInc_Z_Nm/1 -> [VTQR_RDCActiveFEDUInc_Nm]  "VTQR_RDCActiveFEDUInc_Nm"
  [VVMC_ActMaxSlideRate_pct] -> MTQR_AltRDCActiveFEDUInc_Z_Nm/2
  Data Type Conversion/1 -> MTQR_AltRDCActiveFEDUInc_Z_Nm/1
  [VTQR_RDCActiveFEDUInc_Nm] -> Switch/1
  VTQD_RegenTqLimitEn_flg/1 -> [VTQD_RegenTqLimitEn_flg]
  VVMC_ActMaxSlideRate_pct/1 -> [VVMC_ActMaxSlideRate_pct]
  VTQD_PedAccTqEn_flg/1 -> Terminator/1
  Demux/2 -> Switch7/3
  [VTQR_VMCFEDUTqDecSR_Nm] -> Switch7/1
  AND2/1 -> Switch7/2
  [VTQD_RegenTqLimitEn_flg] -> AND2/1
  Switch7/1 -> Gain1/1
  Constant6/1 -> AND2/2
  [VTQR_FEDUWhlTqReqSmoothDelay_Nm] -> VTQR_SPORTFEDURateLimitInc_Nm/4(VTQR_REDUWhlTqReqSmoothDelay_Nm)
  [VDHP_ActAPSPosn_pct] -> VTQR_SPORTFEDURateLimitInc_Nm/1(VDHP_ActAPSPosn_pct)
  [VTQD_RegenMode_enum] -> VTQR_ECOFEDURateLimitInc_Nm/3(VTQD_RegenMode_enum)
  [VTQD_RegenMode_enum] -> VTQR_NORMALFEDURateLimitInc_Nm/3(VTQD_RegenMode_enum)
  [VTQR_FEDUWhlTqReqSmoothDelay_Nm] -> VTQR_ECOFEDURateLimitInc_Nm/4(VTQR_REDUWhlTqReqSmoothDelay_Nm)
  [VTQR_FEDUWhlTqReqSmoothDelay_Nm] -> VTQR_NORMALFEDURateLimitInc_Nm/4(VTQR_FEDUWhlTqReqSmoothDelay_Nm)
  [VTQD_TqTargetShaftSpd_rpm] -> Abs13/1
  [VTQD_RegenMode_enum] -> VTQR_SPORTFEDURateLimitInc_Nm/3(VTQD_RegenMode_enum)
  VTQR_ECOFEDURateLimitInc_Nm/1(VTQR_ECOFEDURateLimitInc_Nm) -> Merge1/3
  [VDHP_ActAPSPosn_pct] -> VTQR_ECOFEDURateLimitInc_Nm/1(VDHP_ActAPSPosn_pct)
  Abs11/1 -> VTQR_SPORTFEDURateLimitInc_Nm/2(VTQD_TqTargetShaftSpd_rpm)  "VTQD_TqTargetShaftSpd_rpm"
  If1/3 -> VTQR_ECOFEDURateLimitInc_Nm/Action
  [VTQD_TqTargetShaftSpd_rpm] -> Abs12/1
  VTQR_NORMALFEDURateLimitInc_Nm/1(VTQR_NORMALFEDURateLimitInc_Nm) -> Merge1/2
  [VTQD_TqTargetShaftSpd_rpm] -> Abs11/1
  VTQR_SPORTFEDURateLimitInc_Nm/1(VTQR_SPORTFEDURateLimitInc_Nm) -> Merge1/4
  If1/4 -> VTQR_SPORTFEDURateLimitInc_Nm/Action
  Abs12/1 -> VTQR_ECOFEDURateLimitInc_Nm/2(VTQD_TqTargetShaftSpd_rpm)  "VTQD_TqTargetShaftSpd_rpm"
  [VDHP_ActAPSPosn_pct] -> VTQR_NORMALFEDURateLimitInc_Nm/1(VDHP_ActAPSPosn_pct)
  If1/2 -> VTQR_NORMALFEDURateLimitInc_Nm/Action
  Abs13/1 -> VTQR_NORMALFEDURateLimitInc_Nm/2(VTQD_TqTargetShaftSpd_rpm)  "VTQD_TqTargetShaftSpd_rpm"
  [VTQR_FrDrModDecLatch_flg] -> Delay4/1
  Constant13/1 -> Mux2/2
  Mux2/1 -> Switch6/3
  Constant10/1 -> Mux2/1
  [VTQD_CreepPrLoadEnable_flg] -> Switch6/2
  Mux1/1 -> Switch6/1
  Switch6/1 -> Switch2/1

== system tqr/TQR/Determine Torque Request/TorqueArbitrament/TorqueSmooth/Limit ==
  input : Inport
  upper_limit : Inport  Port=2
  lower_limit : Inport  Port=3
  MinMax10 : MinMax  Function=max  Inputs=2
  MinMax5 : MinMax  Inputs=2
  out : Outport
  wires:
  lower_limit/1 -> MinMax10/2
  upper_limit/1 -> MinMax5/2
  MinMax10/1 -> out/1
  input/1 -> MinMax5/1
  MinMax5/1 -> MinMax10/1

== system tqr/TQR/Determine Torque Request/TorqueArbitrament/TorqueSmooth/RateLimit ==
  input_raw : Inport
  initial_value : Inport  Port=2
  steptime : Inport  Port=3
  ratelimt_inc : Inport  Port=4
  ratelimt_dec : Inport  Port=5
  MinMax : MinMax  Inputs=2
  MinMax1 : MinMax  Function=max  Inputs=2
  MinMax2 : MinMax  Function=max  Inputs=2
  MinMax3 : MinMax  Inputs=2
  Product : Product  RndMeth=Zero
  Product1 : Product  RndMeth=Zero
  Resettable Delay : Delay  DelayLength=1  InitialConditionSource=Input port
      settings: InputPortMap=u0,p4
  Sum5 : Sum  Inputs=+-
  Sum6 : Sum
  step_time6 : Constant  Value=0  OutDataTypeStr=single
  output : Outport
  wires:
  ratelimt_dec/1 -> Product1/2
  steptime/1 -> Product1/1, Product/2
  Sum5/1 -> MinMax1/1
  [Dec] -> MinMax1/2
  [Inc] -> MinMax/1
  MinMax1/1 -> MinMax/2
  MinMax/1 -> Sum6/1
  input_raw/1 -> Sum5/1
  Sum6/1 -> Resettable Delay/1, output/1
  Resettable Delay/1 -> Sum5/2, Sum6/2
  Product/1 -> MinMax2/1
  Product1/1 -> MinMax3/2
  step_time6/1 -> MinMax2/2, MinMax3/1
  MinMax2/1 -> [Inc]
  MinMax3/1 -> [Dec]
  ratelimt_inc/1 -> Product/1
  initial_value/1 -> Resettable Delay/2

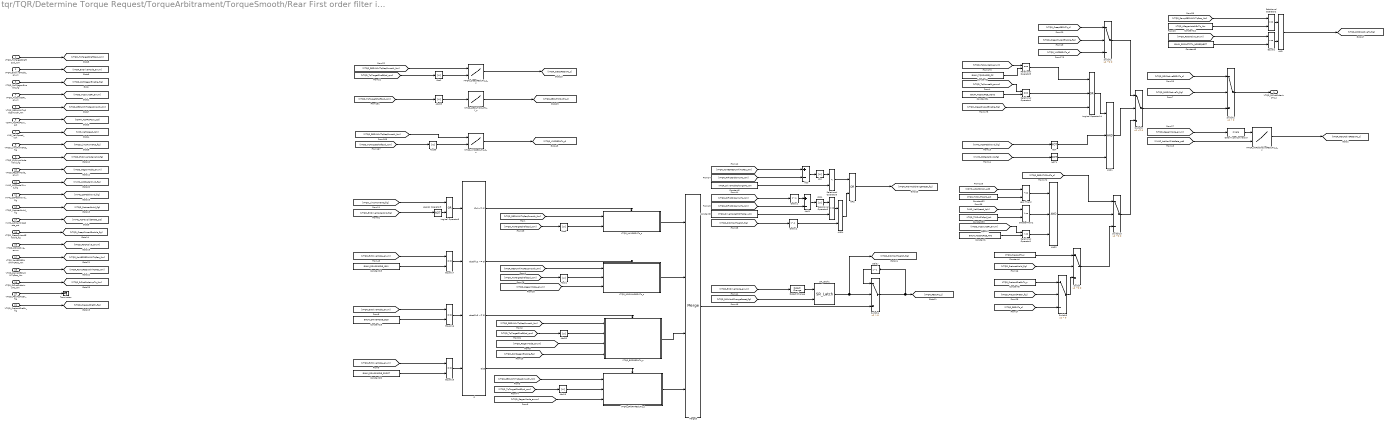
== system tqr/TQR/Determine Torque Request/TorqueArbitrament/TorqueSmooth/Rear First order filter input tau map and determination ==
  VTQD_TqTargetShaftSpd_rpm : Inport
  VTQR_EVDriveMode_enum : Inport  Port=2
  VTQD_RollRegenEnable_flg : Inport  Port=3
  VTQD_TqSourceRr_enum : Inport  Port=4
  VTQR_REDUWhlTqReqSmooth_Nm : Inport  Port=5
  VDHP_ActAPSPosn_pct : Inport  Port=6
  VINP_VehSpeed_kph : Inport  Port=7
  VTQD_LimpHomeAct_flg : Inport  Port=8
  VTQD_EVDriveModeValid_flg : Inport  Port=9
  VTQD_RegenMode_enum : Inport  Port=10
  VVMC_ACCPedalOvrd_flg : Inport  Port=11
  VVMC_CCPedalOvrd_flg : Inport  Port=12
  VTQD_PreLoadHold_flg : Inport  Port=13
  VVMC_ActMaxSlideRate_pct : Inport  Port=14
  VTQD_CreepPrLoadEnable_flg : Inport  Port=15
  VTQD_RDCActive_enum : Inport  Port=16
  VTQR_NoABSREDUWhlTqReq_Nm : Inport  Port=17
  VTQR_RampREDUWhlTqReq_Nm : Inport  Port=18
  VTQR_RrFirstOrderInpTq_Nm : Inport  Port=19
  VTQD_PedAccTqEn_flg : Inport  Port=20
  VTQD_PreLoadPreEn_flg : Inport  Port=21
  AND : Logic  AllPortsSameDT=off  OutDataTypeStr=boolean
  AND1 : Logic  Inputs=3  AllPortsSameDT=off  OutDataTypeStr=boolean
  AND2 : Logic  Inputs=3  AllPortsSameDT=off  OutDataTypeStr=boolean
  AND4 : Logic  AllPortsSameDT=off  OutDataTypeStr=boolean
  Abs{,1,3..4,19..21,33,39} (9 alike) : Abs
  Add : Sum  Inputs=+-
  Add1 : Sum  Inputs=+-
  Constant1 : Constant  Value=ENUM_TQSOURCE_APS
  Constant12 : Constant  Value=KTQR_ARegenLatchEnTq_Nm
  Constant18 : Constant  Value=ENUM_DRIVEMODE_ECO
  Constant19 : Constant  Value=ENUM_DRIVEMODE_NRM
  Constant2 : Constant  Value=KTQR_DriveModeChangeTq_Nm
  Constant20 : Constant  Value=ENUM_DRIVEMODE_SPORT
  Constant3 : Constant  Value=ENUM_TQSOURCE_CC
  Constant32 : Constant  Value=KTQR_TIPOutTsAPS_pct
  Constant33 : Constant  Value=KTQR_TIPOutTsSpd_kph
  Constant34 : Constant  Value=ENUM_TQSOURCE_ADAS
  Constant4 : Constant  Value=KTQR_PreLoadTs_c
  Constant5 : Constant  Value=ENUM_RDCACTSTA_NOREQUEST
  Constant6 : Constant  Value=KTQR_PreLoadPreEnTs_c
  Constant8 : Constant  Value=KTQR_DriveModeCMDTqDev_Nm
  Data Type Conversion : DataTypeConversion  OutDataTypeStr=single
  Delay : Delay  DelayLength=1
  Delay1 : Delay  DelayLength=1
  Delay2 : Delay  DelayLength=1
  Detect Change : simulink/Logic and Bit Operations/Detect Change  vinit=0  OutDataTypeStr=boolean
  Equal16 : RelationalOperator  Operator===  OutDataTypeStr=boolean  RndMeth=Simplest
  Equal17 : RelationalOperator  Operator===  OutDataTypeStr=boolean  RndMeth=Simplest
  Equal19 : RelationalOperator  Operator===  OutDataTypeStr=boolean  RndMeth=Simplest
  Equal2 : RelationalOperator  Operator=~=  OutDataTypeStr=boolean  RndMeth=Simplest
  GreaterThan2 : RelationalOperator  OutDataTypeStr=boolean  RndMeth=Simplest
  If : If  NumInputs=4  IfExpression=u1~= 0  ElseIfExpressions=u2 ~= 0, u3 ~= 0
  Less Than2 : RelationalOperator  Operator=<=  OutDataTypeStr=boolean  RndMeth=Simplest
  Logical Operator14 : Logic  Operator=OR  Inputs=3  AllPortsSameDT=off  OutDataTypeStr=boolean
  Logical Operator8 : Logic  Operator=OR  AllPortsSameDT=off  OutDataTypeStr=boolean
  Logical Operator9 : Logic  Operator=NOT  AllPortsSameDT=off  OutDataTypeStr=boolean
  MTQR_AltRDCActiveREDUTs_Z_c : Lookup_n-D  BreakpointsForDimension1=ATQR_AltRDCActiveREDUTs_Y_enum  BreakpointsForDimension2=ATQR_AltRDCActiveREDUTs_X_pct  Table=MTQR_AltRDCActiveREDUTs_Z_c  TableDataTypeStr=Inherit: Inherit from 'Table data'  ExtrapMethod=Clip  InternalRulePriority=Speed  RndMeth=Simplest  InputSameDT=on
      settings: InputPortMap=u0,u1
  MTQR_CreepREDUTs_Z_c : Lookup_n-D  BreakpointsForDimension1=ATQR_CreepFEDUTs_Y_Nm  BreakpointsForDimension2=ATQR_CreepFEDUTs_X_rpm  Table=MTQR_CreepREDUTs_Z_c  ExtrapMethod=Clip  InternalRulePriority=Speed  RndMeth=Simplest  InputSameDT=on
      settings: InputPortMap=u0,u1
  MTQR_REDUTIPOutTs_Y_c : Lookup_n-D  NumberOfTableDimensions=1  BreakpointsForDimension1=ATQR_FEDUTIPOutTs_X_rpm  Table=MTQR_REDUTIPOutTs_Y_c  ExtrapMethod=Clip  InternalRulePriority=Speed  RndMeth=Simplest  InputSameDT=on
  MTQR_VMCREDUTs_Z_c : Lookup_n-D  BreakpointsForDimension1=ATQR_VMCREDUTs_Y_Nm  BreakpointsForDimension2=ATQR_VMCFEDUTs_X_rpm  Table=MTQR_VMCREDUTs_Z_c  ExtrapMethod=Clip  InternalRulePriority=Speed  RndMeth=Simplest  InputSameDT=on
      settings: InputPortMap=u0,u1
  Merge3 : Merge  Inputs=4
  NOT : Logic  Operator=NOT  AllPortsSameDT=off  OutDataTypeStr=boolean
  NOT1 : Logic  Operator=NOT  AllPortsSameDT=off  OutDataTypeStr=boolean
  OR2 : Logic  Operator=OR  AllPortsSameDT=off  OutDataTypeStr=boolean
  Relational Operator1 : RelationalOperator  Operator=~=  OutDataTypeStr=boolean  RndMeth=Simplest
  Relational Operator2 : RelationalOperator  Operator=<=  OutDataTypeStr=boolean  RndMeth=Simplest
  Relational Operator3 : RelationalOperator  Operator===  OutDataTypeStr=boolean  RndMeth=Simplest
  Relational Operator4 : RelationalOperator  Operator===  OutDataTypeStr=boolean  RndMeth=Simplest
  Relational Operator5 : RelationalOperator  Operator=<  OutDataTypeStr=boolean  RndMeth=Simplest
  Relational Operator6 : RelationalOperator  OutDataTypeStr=boolean  RndMeth=Simplest
  SR_Latch1 : hcu_lib/Basic_Blocks/SR_Latch
  Switch : Switch  Criteria=u2 ~= 0
  Switch1 : Switch  Criteria=u2 ~= 0  Threshold=0.5
  Switch13 : Switch  Criteria=u2 ~= 0
  Switch2 : Switch  Criteria=u2 > Threshold
  Switch3 : Switch  Criteria=u2 ~= 0  Threshold=0.5
  Switch4 : Switch  Criteria=u2 > Threshold
  Switch5 : Switch  Criteria=u2 > Threshold
  Terminator : Terminator
  VTQR_ECOREDUTs_c : Subsystem  AncestorBlock=tqr/TQR/Determine Torque Request/TorqueArbitrament/TorqueSmooth/Front First order filter input tau map and determination/VTQR_ECOFEDUTs_c  TreatAsAtomicUnit=on
  VTQR_LHMREDUTs_c : Subsystem  AncestorBlock=tqr/TQR/Determine Torque Request/TorqueArbitrament/TorqueSmooth/VTQR_LHMREDUTs_c  TreatAsAtomicUnit=on
  VTQR_NORMALREDUTs_c : Subsystem  AncestorBlock=tqr/TQR/Determine Torque Request/TorqueArbitrament/TorqueSmooth/Front First order filter input tau map and determination/VTQR_NORMALFEDUTs_c  TreatAsAtomicUnit=on
  VTQR_SPORTREDUTs_c : Subsystem  AncestorBlock=tqr/TQR/Determine Torque Request/TorqueArbitrament/TorqueSmooth/Front First order filter input tau map and determination/VTQR_SPORTFEDUTs_c  TreatAsAtomicUnit=on
  VTQR_RrFirstOrderInpTs_c : Outport
  wires:
  Abs3/1 -> VTQR_LHMREDUTs_c/2(VTQD_TqTargetShaftSpd_rpm)  "VTQD_TqTargetShaftSpd_rpm"
  VTQR_LHMREDUTs_c/1(VTQR_LHMREDUTs_c) -> Merge3/1
  MTQR_VMCREDUTs_Z_c/1 -> [VTQR_VMCREDUTs_c]  "VTQR_VMCREDUTs_c"
  Equal19/1 -> If/4
  Constant18/1 -> Equal16/2
  Constant19/1 -> Equal17/2
  [VTQD_TqTargetShaftSpd_rpm] -> Abs39/1
  Logical Operator8/1 -> If/1
  Equal16/1 -> If/3
  Equal17/1 -> If/2
  [VTQD_TqTargetShaftSpd_rpm] -> Abs3/1
  [VTQR_EVDriveMode_enum] -> Equal16/1
  Constant20/1 -> Equal19/2
  VTQR_NORMALREDUTs_c/1(VTQR_NORMALREDUTs_c) -> Merge3/2
  [VTQD_EVDriveModeValid_flg] -> Logical Operator9/1
  [VTQR_EVDriveMode_enum] -> Equal19/1
  If/4 -> VTQR_SPORTREDUTs_c/Action
  [VTQR_EVDriveMode_enum] -> Equal17/1
  [VTQD_TqTargetShaftSpd_rpm] -> Abs21/1
  [VTQD_TqTargetShaftSpd_rpm] -> Abs20/1
  [VTQR_REDUWhlTqReqSmooth_Nm] -> VTQR_LHMREDUTs_c/1(VTQR_REDUWhlTqReqSmooth_Nm)
  [VTQD_TqTargetShaftSpd_rpm] -> Abs19/1
  Abs21/1 -> VTQR_NORMALREDUTs_c/2(VTQD_TqTargetShaftSpd_rpm)  "VTQD_TqTargetShaftSpd_rpm"
  If/1 -> VTQR_LHMREDUTs_c/Action
  [VTQR_REDUWhlTqReqSmooth_Nm] -> VTQR_ECOREDUTs_c/1(VTQR_FEDUWhlTqReqSmoothDelay_Nm)
  Abs20/1 -> VTQR_ECOREDUTs_c/2(VTQD_TqTargetShaftSpd_rpm)  "VTQD_TqTargetShaftSpd_rpm"
  [VTQR_REDUWhlTqReqSmooth_Nm] -> VTQR_NORMALREDUTs_c/1(VTQR_FEDUWhlTqReqSmoothDelay_Nm)
  VTQR_SPORTREDUTs_c/1(VTQR_SPORTREDUTs_c) -> Merge3/4
  [VTQD_LimpHomeAct_flg] -> Logical Operator8/1
  VTQR_ECOREDUTs_c/1(VTQR_ECOREDUTs_c) -> Merge3/3
  Logical Operator9/1 -> Logical Operator8/2
  [VTQD_TqTargetShaftSpd_rpm] -> Abs33/1
  Abs33/1 -> MTQR_REDUTIPOutTs_Y_c/1
  MTQR_REDUTIPOutTs_Y_c/1 -> [VTQR_REDUTIPOutTs_c]  "VTQR_REDUTIPOutTs_c"
  VTQR_EVDriveMode_enum/1 -> [VTQR_EVDriveMode_enum]
  VTQD_TqTargetShaftSpd_rpm/1 -> [VTQD_TqTargetShaftSpd_rpm]
  VTQD_TqSourceRr_enum/1 -> [VTQD_TqSourceRr_enum]
  VTQR_REDUWhlTqReqSmooth_Nm/1 -> [VTQR_REDUWhlTqReqSmooth_Nm]
  VTQD_LimpHomeAct_flg/1 -> [VTQD_LimpHomeAct_flg]
  VDHP_ActAPSPosn_pct/1 -> [VDHP_ActAPSPosn_pct]
  VINP_VehSpeed_kph/1 -> [VINP_VehSpeed_kph]
  VTQD_RollRegenEnable_flg/1 -> [VTQD_RollRegenEnable_flg]
  VTQD_EVDriveModeValid_flg/1 -> [VTQD_EVDriveModeValid_flg]
  [VTQD_RegenMode_enum] -> VTQR_NORMALREDUTs_c/3(VTQD_RegenMode_enum)
  [VTQD_RegenMode_enum] -> VTQR_ECOREDUTs_c/3(VTQD_RegenMode_enum)
  [VTQD_RegenMode_enum] -> VTQR_SPORTREDUTs_c/3(VTQD_RegenMode_enum)
  [VTQR_REDUWhlTqReqSmooth_Nm] -> VTQR_SPORTREDUTs_c/1(VTQR_FEDUWhlTqReqSmoothDelay_Nm)
  Abs19/1 -> VTQR_SPORTREDUTs_c/2(VTQD_TqTargetShaftSpd_rpm)  "VTQD_TqTargetShaftSpd_rpm"
  If/3 -> VTQR_ECOREDUTs_c/Action
  If/2 -> VTQR_NORMALREDUTs_c/Action
  VTQD_RegenMode_enum/1 -> [VTQD_RegenMode_enum]
  [VTQD_RollRegenEnable_flg] -> VTQR_ECOREDUTs_c/4(VTQD_RollRegenEnable_flg)
  Abs39/1 -> MTQR_VMCREDUTs_Z_c/2
  [VTQR_REDUWhlTqReqSmooth_Nm] -> MTQR_VMCREDUTs_Z_c/1
  VVMC_ACCPedalOvrd_flg/1 -> [VVMC_ACCPedalOvrd_flg]
  VVMC_CCPedalOvrd_flg/1 -> [VVMC_CCPedalOvrd_flg]
  Constant3/1 -> Relational Operator3/2
  Relational Operator3/1 -> Logical Operator14/1
  [VINP_VehSpeed_kph] -> GreaterThan2/1
  Relational Operator4/1 -> Logical Operator14/2
  Constant34/1 -> Relational Operator4/2
  [VTQD_TqSourceRr_enum] -> Relational Operator4/1
  Less Than2/1 -> AND2/1
  [VTQD_TqSourceRr_enum] -> Relational Operator1/1
  [VTQR_REDUTIPOutTs_c] -> Switch13/1
  AND1/1 -> Switch3/2
  NOT1/1 -> AND1/3
  Switch13/1 -> Switch3/3
  NOT/1 -> AND1/2
  Constant33/1 -> GreaterThan2/2
  GreaterThan2/1 -> AND2/2
  Constant1/1 -> Relational Operator1/2
  Logical Operator14/1 -> AND1/1
  Relational Operator1/1 -> AND2/3
  [VVMC_CCPedalOvrd_flg] -> NOT1/1
  AND2/1 -> Switch13/2
  [VVMC_ACCPedalOvrd_flg] -> NOT/1
  [VTQD_TqSourceRr_enum] -> Relational Operator3/1
  [VDHP_ActAPSPosn_pct] -> Less Than2/1
  Constant32/1 -> Less Than2/2
  Switch2/1 -> VTQR_RrFirstOrderInpTs_c/1  "VTQR_RrFirstOrderInpTs_c"
  [VTQD_PreLoadHold_flg] -> Switch/2
  Constant4/1 -> Switch/1
  Switch/1 -> Switch13/3
  VTQD_PreLoadHold_flg/1 -> [VTQD_PreLoadHold_flg]
  [VTQD_CreepPrLoadEnable_flg] -> Switch1/2
  [VTQR_CreepREDUTs_c] -> Switch1/1
  [VTQR_VMCREDUTs_c] -> Switch1/3
  Switch1/1 -> Switch3/1
  VTQD_CreepPrLoadEnable_flg/1 -> [VTQD_CreepPrLoadEnable_flg]
  Abs1/1 -> MTQR_CreepREDUTs_Z_c/2
  [VTQR_REDUWhlTqReqSmooth_Nm] -> MTQR_CreepREDUTs_Z_c/1
  [VTQD_TqTargetShaftSpd_rpm] -> Abs1/1
  MTQR_CreepREDUTs_Z_c/1 -> [VTQR_CreepREDUTs_c]  "VTQR_CreepREDUTs_c"
  [VTQD_CreepPrLoadEnable_flg] -> Logical Operator14/3
  Constant12/1 -> Relational Operator2/2
  [VTQR_RampREDUWhlTqReq_Nm] -> Relational Operator2/1
  [VTQD_RDCActive_enum] -> Equal2/1
  Equal2/1 -> AND/2
  Constant5/1 -> Equal2/2
  AND/1 -> [VTQR_RrRDCActiveTs_flg]  "VTQR_RrRDCActiveTs_flg"
  Relational Operator2/1 -> AND/1
  [VTQR_RrRDCActiveTs_flg] -> Switch2/2
  Switch3/1 -> Switch2/3
  VTQD_RDCActive_enum/1 -> [VTQD_RDCActive_enum]
  VTQR_NoABSREDUWhlTqReq_Nm/1 -> [VTQR_NoABSREDUWhlTqReq_Nm]
  VTQR_RampREDUWhlTqReq_Nm/1 -> [VTQR_RampREDUWhlTqReq_Nm]
  Add/1 -> Abs/1
  Delay2/1 -> AND4/2
  AND4/1 -> OR2/2
  [VTQR_EVDriveMode_enum] -> Detect Change/1
  Constant2/1 -> Relational Operator5/2
  Delay/1 -> Switch4/1
  Switch4/1 -> [VTQR_REDUTs_c], Delay/1  "VTQR_REDUTs_c"
  Relational Operator6/1 -> AND4/1
  Merge3/1 -> Switch4/3
  SR_Latch1/1 -> Switch4/2, [VTQR_RrDrModTsLatch_flg]  "VTQR_RrDrModLatch_flg"
  Delay1/1 -> Add1/1
  Abs/1 -> Relational Operator5/1
  [VTQR_RrDrModChangeReset_flg] -> SR_Latch1/2
  [VTQR_RrDrModTsLatch_flg] -> Delay2/1
  Detect Change/1 -> SR_Latch1/1
  Constant8/1 -> Relational Operator6/2
  Abs4/1 -> Relational Operator6/1
  OR2/1 -> [VTQR_RrDrModChangeReset_flg]
  Add1/1 -> Abs4/1
  [VTQR_RrFirstOrderInpTq_Nm] -> Delay1/1
  [VTQR_RrFirstOrderInpTq_Nm] -> Add1/2
  [VTQR_RrFirstOrderInpTq_Nm] -> Add/2
  Relational Operator5/1 -> OR2/1
  [VTQR_NoABSREDUWhlTqReq_Nm] -> Add/1
  VTQR_RrFirstOrderInpTq_Nm/1 -> [VTQR_RrFirstOrderInpTq_Nm]
  Data Type Conversion/1 -> MTQR_AltRDCActiveREDUTs_Z_c/1
  MTQR_AltRDCActiveREDUTs_Z_c/1 -> [VTQR_RDCActiveREDUTs_c]  "VTQR_RDCActiveREDUTs_c"
  [VTQD_RegenMode_enum] -> Data Type Conversion/1
  [VTQR_RDCActiveREDUTs_c] -> Switch2/1
  [VVMC_ActMaxSlideRate_pct] -> MTQR_AltRDCActiveREDUTs_Z_c/2
  VTQD_PedAccTqEn_flg/1 -> Terminator/1
  VVMC_ActMaxSlideRate_pct/1 -> [VVMC_ActMaxSlideRate_pct]
  VTQD_PreLoadPreEn_flg/1 -> [VTQD_PreLoadPreEn_flg]
  Switch5/1 -> Switch/3
  [VTQR_REDUTs_c] -> Switch5/3
  [VTQD_PreLoadPreEn_flg] -> Switch5/2
  Constant6/1 -> Switch5/1
